simulink model "Bezier_9g"  (R2015a)
settings: Solver=ode4  StartTime=0.0  StopTime=10.0  FixedStep=5e-3  RelTol=1e-3
settings Model: Creator=Sala6  LastModifiedBy=Jesus

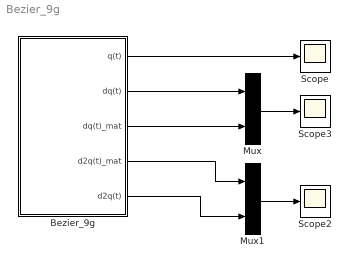
== system Bezier_9g ==
  Bezier_9g : Subsystem  mask{t0=4.8, t1=5.2, q0=4, q1=8}
      mask prompts: t0 "Tiempo de transición"; t1 "Tiempo de transición"; q0 "Posición inicial"; q1 "Posición final"
      mask init:
      | gamma0=126;
      | gamma1=420;
      | gamma2=540;
      | gamma3=315;
      | gamma4=70;
  Mux : Mux  Inputs=2
  Mux1 : Mux  Inputs=2
  Scope : Scope
  Scope2 : Scope
      settings: SaveName=ScopeData2
  Scope3 : Scope
      settings: SaveName=ScopeData3
  wires:
  Bezier_9g/1(q(t)) -> Scope/1
  Bezier_9g/2("dq(t) ") -> Mux/1
  Bezier_9g/3(dq(t)_mat) -> Mux/2
  Mux/1 -> Scope3/1
  Bezier_9g/4(d2q(t)_mat) -> Mux1/1
  Bezier_9g/5(d2q(t)) -> Mux1/2
  Mux1/1 -> Scope2/1

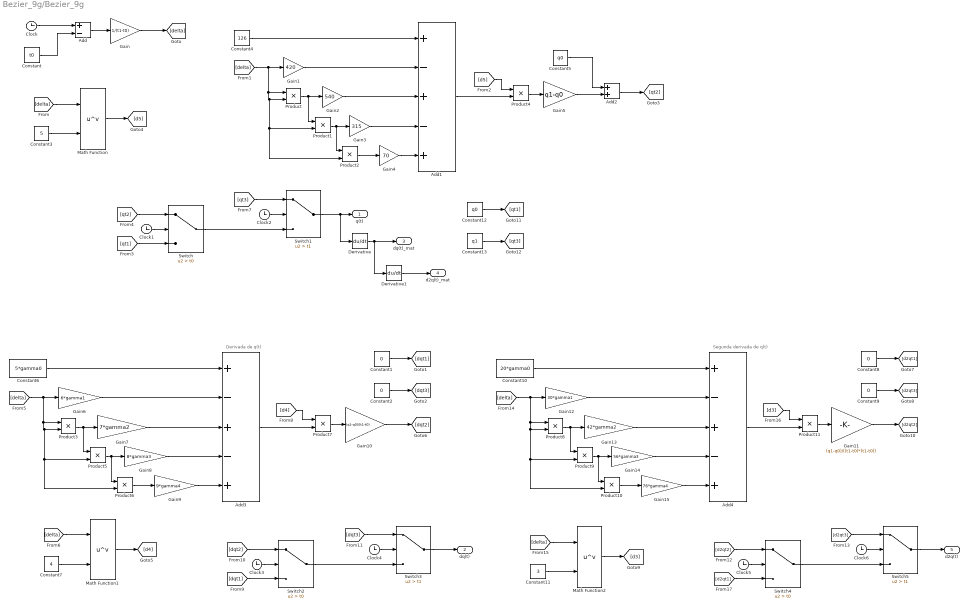
== system Bezier_9g/Bezier_9g ==
  note: Derivada de q(t)
  note: Segunda derivada de q(t)
  Add : Sum  Inputs=+-
  Add1 : Sum  Inputs=+-+-+
  Add2 : Sum
  Add3 : Sum  Inputs=+-+-+
  Add4 : Sum  Inputs=+-+-+
  Clock{,1..6} (7 alike) : Clock
  Constant : Constant  Value=t0
  Constant{1..2,8..9} (4 alike) : Constant  Value=0
  Constant10 : Constant  Value=20*gamma0
  Constant11 : Constant  Value=3
  Constant12 : Constant  Value=q0
  Constant13 : Constant  Value=q1
  Constant3 : Constant  Value=5
  Constant4 : Constant  Value=126
  Constant5 : Constant  Value=q0
  Constant6 : Constant  Value=5*gamma0
  Constant7 : Constant  Value=4
  Derivative : Derivative
  Derivative1 : Derivative
  Gain : Gain  Gain=1/(t1-t0)
  Gain1 : Gain  Gain=420
  Gain10 : Gain  Gain=(q1-q0)/(t1-t0)
  Gain11 : Gain  Gain=(q1-q0)/((t1-t0)*(t1-t0))
  Gain12 : Gain  Gain=30*gamma1
  Gain13 : Gain  Gain=42*gamma2
  Gain14 : Gain  Gain=56*gamma3
  Gain15 : Gain  Gain=76*gamma4
  Gain2 : Gain  Gain=540
  Gain3 : Gain  Gain=315
  Gain4 : Gain  Gain=70
  Gain5 : Gain  Gain=q1-q0
  Gain6 : Gain  Gain=6*gamma1
  Gain7 : Gain  Gain=7*gamma2
  Gain8 : Gain  Gain=8*gamma3
  Gain9 : Gain  Gain=9*gamma4
  Math Function : Math  Operator=pow  SaturateOnIntegerOverflow=on
  Math Function1 : Math  Operator=pow  SaturateOnIntegerOverflow=on
  Math Function2 : Math  Operator=pow  SaturateOnIntegerOverflow=on
  Product{,1..11} (12 alike) : Product
  Switch : Switch  Criteria=u2 > Threshold  Threshold=t0
  Switch1 : Switch  Criteria=u2 > Threshold  Threshold=t1
  Switch2 : Switch  Criteria=u2 > Threshold  Threshold=t0
  Switch3 : Switch  Criteria=u2 > Threshold  Threshold=t1
  Switch4 : Switch  Criteria=u2 > Threshold  Threshold=t0
  Switch5 : Switch  Criteria=u2 > Threshold  Threshold=t1
  q(t) : Outport
  "dq(t) " : Outport  Port=2
  dq(t)_mat : Outport  Port=3
  d2q(t)_mat : Outport  Port=4
  d2q(t) : Outport  Port=5
  wires:
  Constant/1 -> Add/2
  Gain/1 -> [delta]
  Add/1 -> Gain/1
  Constant2/1 -> [dqt3]
  Constant1/1 -> [dqt1]
  [delta] -> Math Function/1
  Clock/1 -> Add/1
  Constant3/1 -> Math Function/2
  Product2/1 -> Gain4/1
  Product1/1 -> Product2/1, Gain3/1
  Add1/1 -> Product4/2
  [delta] -> Product2/2, Product1/2, Product/2, Product/1, Gain1/1
  Product/1 -> Product1/1, Gain2/1
  Gain1/1 -> Add1/2
  Constant4/1 -> Add1/1
  Gain3/1 -> Add1/4
  Gain4/1 -> Add1/5
  Gain2/1 -> Add1/3
  [d5] -> Product4/1
  Add2/1 -> [qt2]
  Constant5/1 -> Add2/1
  Product4/1 -> Gain5/1
  Clock1/1 -> Switch/2
  [qt3] -> Switch1/1
  Clock2/1 -> Switch1/2
  Gain5/1 -> Add2/2
  [qt1] -> Switch/3
  [qt2] -> Switch/1
  Math Function/1 -> [d5]
  Switch/1 -> Switch1/3
  Switch1/1 -> Derivative/1, q(t)/1
  Derivative/1 -> Derivative1/1, dq(t)_mat/1
  Derivative1/1 -> d2q(t)_mat/1
  Product6/1 -> Gain9/1
  Product5/1 -> Gain8/1, Product6/1
  [delta] -> Gain6/1, Product3/1, Product3/2, Product5/2, Product6/2
  Product3/1 -> Gain7/1, Product5/1
  Gain6/1 -> Add3/2
  Constant6/1 -> Add3/1
  Gain8/1 -> Add3/4
  Gain9/1 -> Add3/5
  Gain7/1 -> Add3/3
  [delta] -> Math Function1/1
  Constant7/1 -> Math Function1/2
  Math Function1/1 -> [d4]
  Add3/1 -> Product7/2
  [d4] -> Product7/1
  Product7/1 -> Gain10/1
  Gain10/1 -> [dqt2]
  Clock3/1 -> Switch2/2
  [dqt3] -> Switch3/1
  Clock4/1 -> Switch3/2
  [dqt1] -> Switch2/3
  [dqt2] -> Switch2/1
  Switch2/1 -> Switch3/3
  Switch3/1 -> "dq(t) "/1
  Constant9/1 -> [d2qt3]
  Constant8/1 -> [d2qt1]
  Product10/1 -> Gain15/1
  Product9/1 -> Product10/1, Gain14/1
  [delta] -> Product10/2, Product9/2, Product8/2, Product8/1, Gain12/1
  Product8/1 -> Product9/1, Gain13/1
  Gain12/1 -> Add4/2
  Constant10/1 -> Add4/1
  Gain14/1 -> Add4/4
  Gain15/1 -> Add4/5
  Gain13/1 -> Add4/3
  [delta] -> Math Function2/1
  Constant11/1 -> Math Function2/2
  Math Function2/1 -> [d3]
  Add4/1 -> Product11/2
  [d3] -> Product11/1
  Product11/1 -> Gain11/1
  Gain11/1 -> [d2qt2]
  Clock5/1 -> Switch4/2
  [d2qt3] -> Switch5/1
  Clock6/1 -> Switch5/2
  [d2qt1] -> Switch4/3
  [d2qt2] -> Switch4/1
  Switch4/1 -> Switch5/3
  Switch5/1 -> d2q(t)/1
  Constant13/1 -> [qt3]
  Constant12/1 -> [qt1]
